simulink model "ModeSelectorTest"  (R2020b)
settings: Solver=VariableStepAuto  StartTime=0.0  StopTime=1.0  RelTol=1e-3
settings Model: Creator=tyevans  LastModifiedBy=tyevans

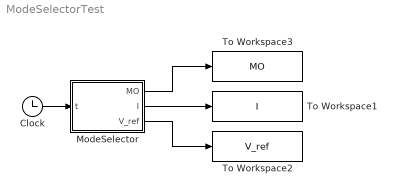
== system ModeSelectorTest ==
  Clock : Clock
  ModeSelector : MATLAB Function  TreatAsAtomicUnit=on
  To Workspace1 : ToWorkspace  VariableName=I  SampleTime=-1
  To Workspace2 : ToWorkspace  VariableName=V_ref  SampleTime=-1
  To Workspace3 : ToWorkspace  VariableName=MO  SampleTime=-1
  wires:
  Clock/1 -> ModeSelector/1(t)
  ModeSelector/2(I) -> To Workspace1/1
  ModeSelector/3(V_ref) -> To Workspace2/1
  ModeSelector/1(MO) -> To Workspace3/1

== matlab function ModeSelectorTest/ModeSelector ==
  data: t input; MO output; I output; V_ref output; SIM parameter
function [MO,I,V_ref] = fcn(t, SIM)
% Initialize Outputs Data Types
MO    = 1;
I     = 0.0;
V_ref = 0.0;

% Call Matlab Function
coder.extrinsic('myMode');
[MO,I,V_ref] = myMode(t,SIM);
end
